simulink library "shared6dofsys"  (R2020a)
settings: Solver=ode45  StartTime=0.0  StopTime=10.0  RelTol=1e-3
values from neighbouring files (symbols this model uses):
  mass_0 = 33296    [Final_Project_EEM_SIM_init_params.m]
undefined symbols (not defined in the file or in its folder): aMode, e0_0, e1_0, e2_0, e3_0, eul_0, inertia, k_quat, mass_e, mass_f
libraries: sharedtransform x4, sharedutil x2, shareddyn x1
Description:
  | Aerospace Blockset Library: 6DoF support library
settings Model: FPTRunName=Active  ModifiedByFormat=The MathWorks, Inc.  ExtModeAutoUpdateStatusClock=off  Creator=The MathWorks, Inc.  LastModifiedBy=The MathWorks, Inc.
settings DataIOCC: LimitDataPoints=on  SaveFormat=Array  SignalLoggingSaveFormat=ModelDataLogs  ReturnWorkspaceOutputs=off
settings OptimizationCC: BlockReduction=off  BooleanDataType=off  ExpressionDepthLimit=2147483647  EfficientMapNaN2IntZero=off  LifeSpan=inf
settings DebuggingCC: SaveWithParameterizedLinksMsg=none  UnderspecifiedInitializationDetection=Classic  MergeDetectMultiDrivingBlocksExec=none  SignalResolutionControl=TryResolveAllWithWarning  FcnCallInpInsideContextMsg=warning  StateNameClashWarn=warning  SFUnexpectedBacktrackingDiag=warning  SFNoUnconditionalDefaultTransitionDiag=warning  SFExecutionAtInitializationDiag=none  ArithmeticOperatorsInVariantConditions=warning
settings HardwareCC: ProdBitPerPointer=32  ProdBitPerSizeT=32  ProdBitPerPtrDiffT=32  ProdLargestAtomicFloat=None  ProdIntDivRoundTo=Undefined  ProdEndianess=Unspecified  ProdWordSize=32  ProdHWDeviceType=32-bit Generic  TargetUnknown=on
settings ModelReferenceCC: PropagateSignalLabelsOutOfModel=off
settings SFSimCC: SimUseLocalCustomCode=off  CustomCodeUndefinedFunction=UseInterfaceOnly
settings RTWCC: RTWUseLocalCustomCode=off
settings CodeAppCC: StateflowObjectComments=on
settings GRTTargetCC: TargetLangStandard=C89/C90 (ANSI)  CombineOutputUpdateFcns=off  GRTInterface=on
settings ConfigComp: CovMetricSettings=dw  CovHtmlReporting=on  CovSaveCumulativeToWorkspaceVar=on  CovSaveSingleToWorkspaceVar=on  CovShowResultsExplorer=off  CovExternalEMLEnable=off

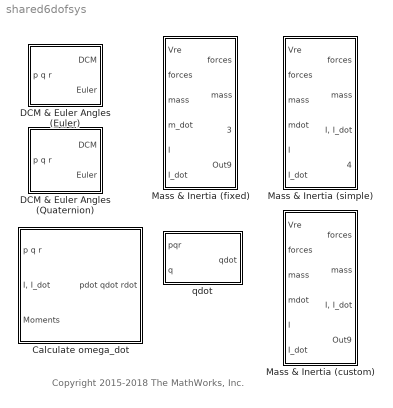
== system shared6dofsys ==
  note: Copyright 2015-2018 The MathWorks, Inc.
  Calculate omega_dot : Subsystem  mask{aMode=aMode}
      mask init:
      | if aerosharedtest(gcb)
      |     aerosharedicon('shared');
      | else
      |     sharedautoicon('shared');
      | end
  DCM & Euler Angles (Euler) : Subsystem  mask(DCM & Euler Angles (Euler)){aMode=aMode}
      mask init:
      | if aerosharedtest(gcb)
      |     aerosharedicon('shared');
      | else
      |     sharedautoicon('shared');
      | end
  DCM & Euler Angles (Quaternion) : Subsystem  mask(DCM & Euler Angles (Quaternion)){aMode=aMode}
      mask init:
      | if aerosharedtest(gcb)
      |     aerosharedicon('shared');
      | else
      |     sharedautoicon('shared');
      | end
  Mass & Inertia (custom) : Subsystem  mask(Mass & Inertia (custom)){aMode=aMode}
      mask init:
      | if aerosharedtest(gcb)
      |     aerosharedicon('shared');
      | else
      |     sharedautoicon('shared');
      | end
  Mass & Inertia (fixed) : Subsystem  mask(Mass & Inertia (fixed)){aMode=aMode}
      mask init:
      | if aerosharedtest(gcb)
      |     aerosharedicon('shared');
      | else
      |     sharedautoicon('shared');
      | end
  Mass & Inertia (simple) : Subsystem  mask(Mass & Inertia (simple)){aMode=aMode}
      mask init:
      | if aerosharedtest(gcb)
      |     aerosharedicon('shared');
      | else
      |     sharedautoicon('shared');
      | end
  qdot : Subsystem  mask{aMode=aMode}
      mask init:
      | if aerosharedtest(gcb)
      |     aerosharedicon('shared');
      | else
      |     sharedautoicon('shared');
      | end

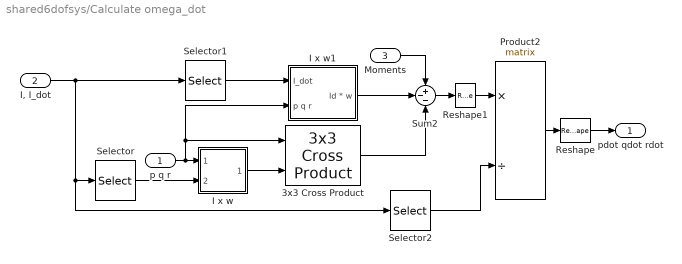
== system shared6dofsys/Calculate omega_dot ==
  p q r : Inport
  "I, I_dot" : Inport  Port=2
  Moments : Inport  Port=3
  3x3 Cross Product : sharedutil/3x3 Cross Product  aMode=aMode
      settings: SourceProductBaseCode=AE,PW,MT,VE,VP
  I x w : Subsystem
  I x w1 : Subsystem
  Product2 : Product  Inputs=*/  Multiplication=Matrix(*)  SaturateOnIntegerOverflow=on  OutDataTypeStr=Inherit: Same as first input
  Reshape : Reshape
  Reshape1 : Reshape  OutputDimensionality=Row vector (2-D)
  Selector : Selector  NumberOfDimensions=2  InputPortWidth=2  IndexOptions=Index vector (dialog),Select all  Indices=1:3,-1  OutputSizes=1
  Selector1 : Selector  NumberOfDimensions=2  InputPortWidth=2  IndexOptions=Index vector (dialog),Select all  Indices=4:6,-1  OutputSizes=1
  Selector2 : Selector  NumberOfDimensions=2  InputPortWidth=2  IndexOptions=Index vector (dialog),Select all  Indices=1:3,-1  OutputSizes=1
  Sum2 : Sum  Inputs=+--  SaturateOnIntegerOverflow=on
  pdot qdot rdot : Outport  VectorParamsAs1DForOutWhenUnconnected=off
  wires:
  Reshape/1 -> pdot qdot rdot/1
  Selector/1 -> I x w/2(Inertia)
  Selector2/1 -> Product2/2
  "I, I_dot"/1 -> Selector/1, Selector2/1, Selector1/1
  p q r/1 -> I x w/1(p q r), 3x3 Cross Product/1, I x w1/2(p q r)
  Product2/1 -> Reshape/1
  Sum2/1 -> Reshape1/1
  Moments/1 -> Sum2/1
  I x w1/1(Id * w) -> Sum2/2
  Selector1/1 -> I x w1/1(I_dot)
  3x3 Cross Product/1 -> Sum2/3
  I x w/1(I * w) -> 3x3 Cross Product/2
  Reshape1/1 -> Product2/1

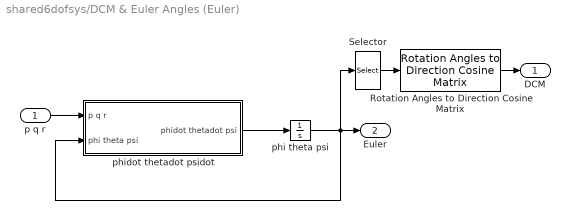
== system shared6dofsys/DCM & Euler Angles (Euler) ==
  "p q r " : Inport
  Rotation Angles to Direction Cosine Matrix : sharedtransform/Rotation Angles to Direction Cosine Matrix  rotationOrder=ZYX  aMode=aMode
      settings: SourceProductBaseCode=AE,PW,MT,VE,VP
  Selector : Selector  InputPortWidth=3  IndexOptions=Index vector (dialog)  Indices=[3 2 1]  OutputSizes=1
  phi theta psi : Integrator  InitialCondition=eul_0  WrapState=on  ContinuousStateAttributes=eul_statename
  phidot thetadot psidot : Subsystem
  DCM : Outport  VectorParamsAs1DForOutWhenUnconnected=off
  Euler : Outport  Port=2  VectorParamsAs1DForOutWhenUnconnected=off
  wires:
  Rotation Angles to Direction Cosine Matrix/1 -> DCM/1
  "p q r "/1 -> phidot thetadot psidot/1(p q r)
  phidot thetadot psidot/1(phidot thetadot psi) -> phi theta psi/1
  phi theta psi/1 -> Euler/1, phidot thetadot psidot/2(phi theta psi), Selector/1
  Selector/1 -> Rotation Angles to Direction Cosine Matrix/1

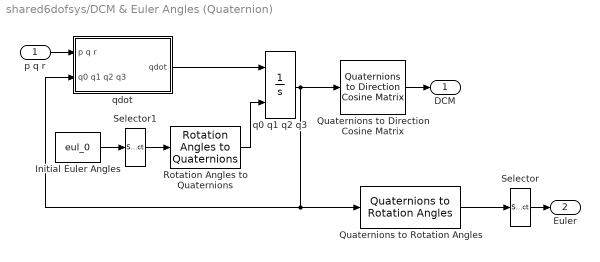
== system shared6dofsys/DCM & Euler Angles (Quaternion) ==
  p q r : Inport
  Initial Euler Angles : Constant  Value=eul_0
  Quaternions to Direction Cosine Matrix : sharedtransform/Quaternions to  Direction Cosine Matrix  aMode=aMode
      settings: SourceProductBaseCode=AE,PW,MT,VE,VP
  Quaternions to Rotation Angles : sharedtransform/Quaternions to Rotation Angles  rotationOrder=ZYX  aMode=aMode
      settings: SourceProductBaseCode=AE,PW,MT,VE,VP
  Rotation Angles to Quaternions : sharedtransform/Rotation Angles to Quaternions  rotationOrder=ZYX  aMode=aMode
      settings: SourceProductBaseCode=AE,PW,MT,VE,VP
  Selector : Selector  InputPortWidth=3  IndexOptions=Index vector (dialog)  Indices=[3 2 1]  OutputSizes=1
  Selector1 : Selector  InputPortWidth=3  IndexOptions=Index vector (dialog)  Indices=[3 2 1]  OutputSizes=1
  q0 q1 q2 q3 : Integrator  InitialConditionSource=external  InitialCondition=[e0_0 e1_0 e2_0 e3_0]  ContinuousStateAttributes=quat_statename
  qdot : Subsystem
  DCM : Outport  VectorParamsAs1DForOutWhenUnconnected=off
  Euler : Outport  Port=2  VectorParamsAs1DForOutWhenUnconnected=off
  wires:
  qdot/1(qdot) -> q0 q1 q2 q3/1
  q0 q1 q2 q3/1 -> Quaternions to Direction Cosine Matrix/1, Quaternions to Rotation Angles/1, qdot/2(q0 q1 q2 q3)
  Rotation Angles to Quaternions/1 -> q0 q1 q2 q3/2
  Initial Euler Angles/1 -> Selector1/1
  p q r/1 -> qdot/1(p q r)
  Quaternions to Direction Cosine Matrix/1 -> DCM/1
  Quaternions to Rotation Angles/1 -> Selector/1
  Selector/1 -> Euler/1
  Selector1/1 -> Rotation Angles to Quaternions/1

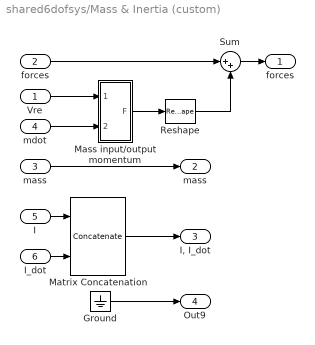
== system shared6dofsys/Mass & Inertia (custom) ==
  Vre : Inport
  forces : Inport  Port=2
  "mass " : Inport  Port=3
  mdot : Inport  Port=4
  I : Inport  Port=5
  I_dot : Inport  Port=6
  Ground : Ground
  Mass input/output momentum : Subsystem
  Matrix Concatenation : Concatenate  Mode=Multidimensional array
  Reshape : Reshape
  Sum : Sum  Inputs=|++  SaturateOnIntegerOverflow=on
  "forces " : Outport  PortDimensions=3  VectorParamsAs1DForOutWhenUnconnected=off
  mass : Outport  Port=2  VectorParamsAs1DForOutWhenUnconnected=off
  "I, I_dot " : Outport  Port=3  VectorParamsAs1DForOutWhenUnconnected=off
  Out9 : Outport  Port=4  VectorParamsAs1DForOutWhenUnconnected=off
  wires:
  Ground/1 -> Out9/1
  I/1 -> Matrix Concatenation/1
  "mass "/1 -> mass/1
  Matrix Concatenation/1 -> "I, I_dot "/1
  I_dot/1 -> Matrix Concatenation/2
  forces/1 -> Sum/1
  Sum/1 -> "forces "/1
  Mass input/output momentum/1(F) -> Reshape/1
  Vre/1 -> Mass input/output momentum/1(Vre)
  mdot/1 -> Mass input/output momentum/2(mdot)
  Reshape/1 -> Sum/2

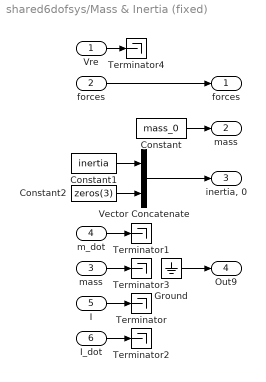
== system shared6dofsys/Mass & Inertia (fixed) ==
  Vre : Inport
  forces : Inport  Port=2
  "mass " : Inport  Port=3
  m_dot : Inport  Port=4  OutDataTypeStr=double
  I : Inport  Port=5  OutDataTypeStr=double
  I_dot : Inport  Port=6  OutDataTypeStr=double
  Constant : Constant  Value=mass_0  OutDataTypeStr=Inherit: Inherit via back propagation
  Constant1 : Constant  Value=inertia  OutDataTypeStr=Inherit: Inherit via back propagation
  Constant2 : Constant  Value=zeros(3)
  Ground : Ground
  Terminator{,1..4} (5 alike) : Terminator
  Vector Concatenate : Concatenate  Mode=Multidimensional array
  "forces " : Outport  VectorParamsAs1DForOutWhenUnconnected=off
  mass : Outport  Port=2  VectorParamsAs1DForOutWhenUnconnected=off
  "inertia, 0" : Outport  Port=3  VectorParamsAs1DForOutWhenUnconnected=off
  Out9 : Outport  Port=4  VectorParamsAs1DForOutWhenUnconnected=off
  wires:
  Constant/1 -> mass/1
  Ground/1 -> Out9/1
  I/1 -> Terminator/1
  m_dot/1 -> Terminator1/1
  I_dot/1 -> Terminator2/1
  "mass "/1 -> Terminator3/1
  forces/1 -> "forces "/1
  Vre/1 -> Terminator4/1
  Constant1/1 -> Vector Concatenate/1
  Constant2/1 -> Vector Concatenate/2
  Vector Concatenate/1 -> "inertia, 0"/1

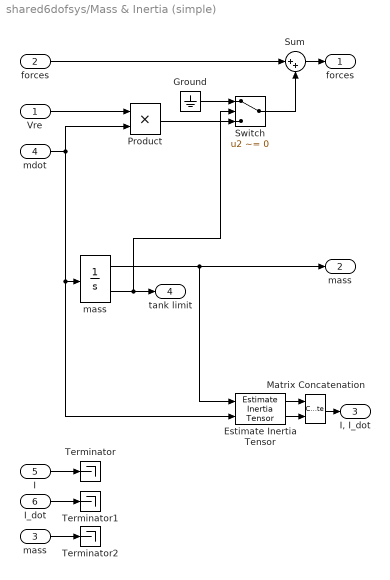
== system shared6dofsys/Mass & Inertia (simple) ==
  Vre : Inport
  forces : Inport  Port=2
  "mass " : Inport  Port=3
  mdot : Inport  Port=4
  I : Inport  Port=5  OutDataTypeStr=double
  I_dot : Inport  Port=6  OutDataTypeStr=double
  Estimate Inertia Tensor : shareddyn/Estimate Inertia Tensor  fmass=mass_f  emass=mass_e  fI=inertia_f  eI=inertia_e  aMode=aMode
      settings: SourceProductBaseCode=AE,PW,MT,VE,VP
  Ground : Ground
  Matrix Concatenation : Concatenate  Mode=Multidimensional array
  Product : Product
  Sum : Sum  Inputs=|++  SaturateOnIntegerOverflow=on
  Switch : Switch  Criteria=u2 ~= 0
  Terminator : Terminator
  Terminator1 : Terminator
  Terminator2 : Terminator
  "mass  " : Integrator  InitialCondition=mass_0  LimitOutput=on  UpperSaturationLimit=mass_f  LowerSaturationLimit=mass_e  ShowSaturationPort=on  ContinuousStateAttributes=mass_statename
  "forces " : Outport  PortDimensions=3  VectorParamsAs1DForOutWhenUnconnected=off
  mass : Outport  Port=2  VectorParamsAs1DForOutWhenUnconnected=off
  "I, I_dot" : Outport  Port=3  VectorParamsAs1DForOutWhenUnconnected=off
  tank limit : Outport  Port=4  VectorParamsAs1DForOutWhenUnconnected=off
  wires:
  "mass  "/2 -> Switch/2, tank limit/1
  "mass  "/1 -> Estimate Inertia Tensor/1, mass/1
  mdot/1 -> Product/2, Estimate Inertia Tensor/2, "mass  "/1
  Estimate Inertia Tensor/1 -> Matrix Concatenation/1
  I/1 -> Terminator/1
  Estimate Inertia Tensor/2 -> Matrix Concatenation/2
  Matrix Concatenation/1 -> "I, I_dot"/1
  I_dot/1 -> Terminator1/1
  "mass "/1 -> Terminator2/1
  forces/1 -> Sum/1
  Sum/1 -> "forces "/1
  Switch/1 -> Sum/2
  Vre/1 -> Product/1
  Ground/1 -> Switch/1
  Product/1 -> Switch/3

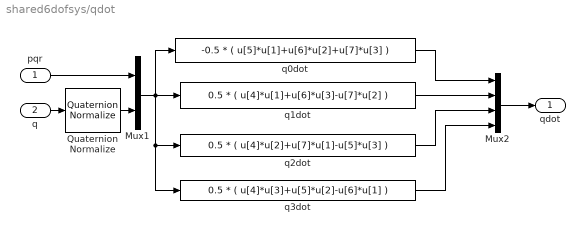
== system shared6dofsys/qdot ==
  pqr : Inport
  q : Inport  Port=2
  Mux1 : Mux  Inputs=[3 4]
  Mux2 : Mux
  Quaternion Normalize : sharedutil/Quaternion Normalize  aMode=aMode
      settings: SourceProductBaseCode=AE,PW,MT,VE,VP
  q0dot : Fcn  Expr=-0.5 * ( u[5]*u[1]+u[6]*u[2]+u[7]*u[3] )
  q1dot : Fcn  Expr=0.5 * ( u[4]*u[1]+u[6]*u[3]-u[7]*u[2] )
  q2dot : Fcn  Expr=0.5 * ( u[4]*u[2]+u[7]*u[1]-u[5]*u[3] )
  q3dot : Fcn  Expr=0.5 * ( u[4]*u[3]+u[5]*u[2]-u[6]*u[1] )
  qdot : Outport  InitialOutput=0  VectorParamsAs1DForOutWhenUnconnected=off
  wires:
  Quaternion Normalize/1 -> Mux1/2
  q/1 -> Quaternion Normalize/1
  q3dot/1 -> Mux2/4
  Mux1/1 -> q1dot/1, q0dot/1, q3dot/1, q2dot/1
  q2dot/1 -> Mux2/3
  q1dot/1 -> Mux2/2
  q0dot/1 -> Mux2/1
  Mux2/1 -> qdot/1
  pqr/1 -> Mux1/1

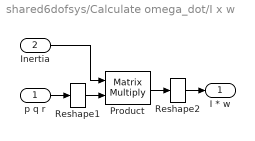
== system shared6dofsys/Calculate omega_dot/I x w ==
  p q r : Inport
  Inertia : Inport  Port=2
  Product : Product  Multiplication=Matrix(*)  InputSameDT=on  SaturateOnIntegerOverflow=on  OutDataTypeStr=Inherit: Same as first input
  Reshape1 : Reshape  OutputDimensionality=Column vector (2-D)
  Reshape2 : Reshape
  I * w : Outport  VectorParamsAs1DForOutWhenUnconnected=off
  wires:
  Product/1 -> Reshape2/1
  Inertia/1 -> Product/1
  p q r/1 -> Reshape1/1
  Reshape1/1 -> Product/2
  Reshape2/1 -> I * w/1

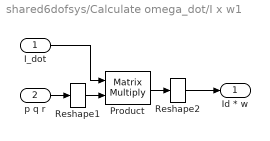
== system shared6dofsys/Calculate omega_dot/I x w1 ==
  I_dot : Inport
  p q r : Inport  Port=2
  Product : Product  Multiplication=Matrix(*)  InputSameDT=on  SaturateOnIntegerOverflow=on  OutDataTypeStr=Inherit: Same as first input
  Reshape1 : Reshape  OutputDimensionality=Column vector (2-D)
  Reshape2 : Reshape
  Id * w : Outport  VectorParamsAs1DForOutWhenUnconnected=off
  wires:
  p q r/1 -> Reshape1/1
  I_dot/1 -> Product/1
  Product/1 -> Reshape2/1
  Reshape1/1 -> Product/2
  Reshape2/1 -> Id * w/1

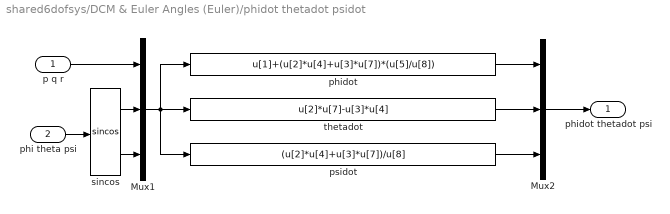
== system shared6dofsys/DCM & Euler Angles (Euler)/phidot thetadot psidot ==
  p q r : Inport
  phi theta psi : Inport  Port=2
  Mux1 : Mux  Inputs=[3 3 3]
  Mux2 : Mux  Inputs=3
  phidot : Fcn  Expr=u[1]+(u[2]*u[4]+u[3]*u[7])*(u[5]/u[8])
  psidot : Fcn  Expr=(u[2]*u[4]+u[3]*u[7])/u[8]
  sincos : Trigonometry  Operator=sincos
  thetadot : Fcn  Expr=u[2]*u[7]-u[3]*u[4]
  phidot thetadot psi : Outport  InitialOutput=0  VectorParamsAs1DForOutWhenUnconnected=off
  wires:
  sincos/2 -> Mux1/3
  sincos/1 -> Mux1/2
  Mux2/1 -> phidot thetadot psi/1
  phidot/1 -> Mux2/1
  thetadot/1 -> Mux2/2
  psidot/1 -> Mux2/3
  phi theta psi/1 -> sincos/1
  p q r/1 -> Mux1/1
  Mux1/1 -> thetadot/1, phidot/1, psidot/1

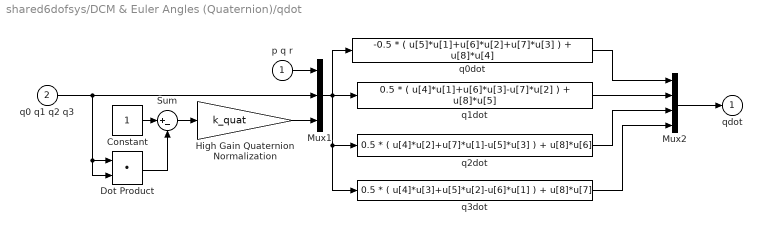
== system shared6dofsys/DCM & Euler Angles (Quaternion)/qdot ==
  p q r : Inport
  q0 q1 q2 q3 : Inport  Port=2
  Constant : Constant
  Dot Product : DotProduct  OutDataTypeStr=Inherit: Inherit via internal rule
  High Gain Quaternion Normalization : Gain  Gain=k_quat  SaturateOnIntegerOverflow=on  OutDataTypeStr=Inherit: Same as input  ParamDataTypeStr=Inherit: Same as input
  Mux1 : Mux  Inputs=[3 4 1]
  Mux2 : Mux
  Sum : Sum  Inputs=|+-  InputSameDT=on  SaturateOnIntegerOverflow=on  OutDataTypeStr=Inherit: Same as first input
  q0dot : Fcn  Expr=-0.5 * ( u[5]*u[1]+u[6]*u[2]+u[7]*u[3] ) + u[8]*u[4]
  q1dot : Fcn  Expr=0.5 * ( u[4]*u[1]+u[6]*u[3]-u[7]*u[2] ) + u[8]*u[5]
  q2dot : Fcn  Expr=0.5 * ( u[4]*u[2]+u[7]*u[1]-u[5]*u[3] ) + u[8]*u[6]
  q3dot : Fcn  Expr=0.5 * ( u[4]*u[3]+u[5]*u[2]-u[6]*u[1] ) + u[8]*u[7]
  qdot : Outport  InitialOutput=0  VectorParamsAs1DForOutWhenUnconnected=off
  wires:
  q0 q1 q2 q3/1 -> Mux1/2, Dot Product/2, Dot Product/1
  q3dot/1 -> Mux2/4
  Mux1/1 -> q1dot/1, q0dot/1, q3dot/1, q2dot/1
  q2dot/1 -> Mux2/3
  q1dot/1 -> Mux2/2
  q0dot/1 -> Mux2/1
  Mux2/1 -> qdot/1
  Constant/1 -> Sum/1
  Sum/1 -> High Gain Quaternion Normalization/1
  High Gain Quaternion Normalization/1 -> Mux1/3
  Dot Product/1 -> Sum/2
  p q r/1 -> Mux1/1

== system shared6dofsys/Mass & Inertia (custom)/Mass input//output momentum ==
  Vre : Inport
  mdot : Inport  Port=2
  For Each Subsystem : Subsystem  TreatAsAtomicUnit=on
  Sum of Elements : Sum  Inputs=+  CollapseMode=Specified dimension  CollapseDim=2
  F : Outport  VectorParamsAs1DForOutWhenUnconnected=off
  wires:
  mdot/1 -> For Each Subsystem/1(mdot)
  Vre/1 -> For Each Subsystem/2(Vre)
  For Each Subsystem/1(F) -> Sum of Elements/1
  Sum of Elements/1 -> F/1

== system shared6dofsys/Mass & Inertia (custom)/Mass input//output momentum/For Each Subsystem ==
  mdot : Inport  Partition=on  PartitionDimension=1  PartitionWidth=1  PartitionOffset=0
  Vre : Inport  Port=2  Partition=on  PartitionDimension=1  PartitionWidth=3  PartitionOffset=0
  For Each : ForEach  DisableCoverage=on
  Product : Product
  F : Outport  ConcatenationDimension=2  VectorParamsAs1DForOutWhenUnconnected=off
  wires:
  mdot/1 -> Product/1
  Vre/1 -> Product/2
  Product/1 -> F/1
